simulink model "MPPCMcontrol"  (R2021a)
settings: Solver=FixedStepDiscrete  StartTime=0.0  StopTime=0.0015  FixedStep=2.5e-8  RelTol=1e-3
libraries: modelsimlib x1
settings Model: Creator=xiang  LastModifiedBy=xiang

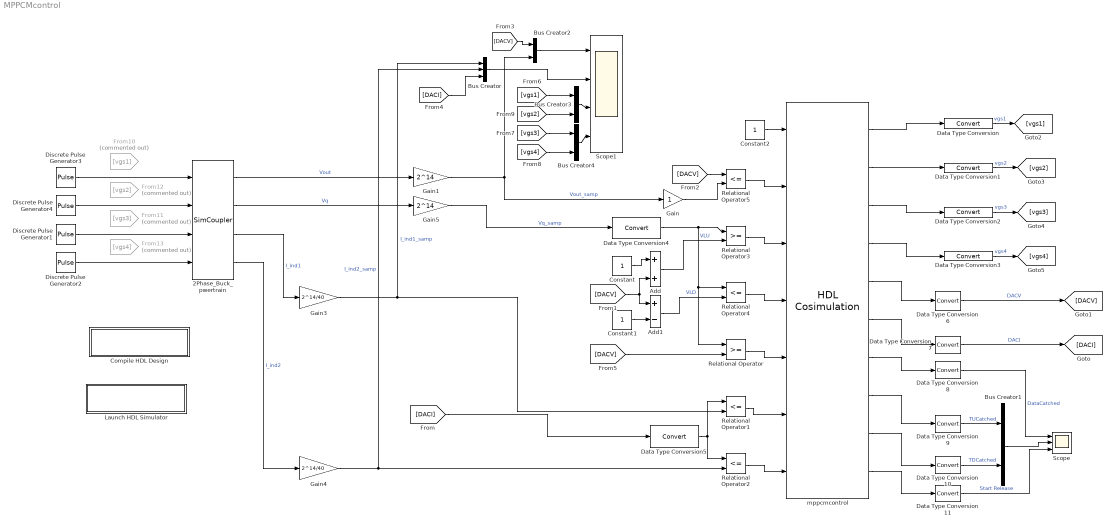
== system MPPCMcontrol ==
  2Phase_Buck_pwertrain : S-Function  FunctionName=SimCoupler  Parameters='C:\Users\xiang\Documents\PSIM\AVP_Simulink_cosim\2Phase_Buck_pwertrain.psimsch;flag_interpolation=0'  SFunctionDeploymentMode=off  EnableBusSupport=off
      mask init:
      | c=[0:10:360]*pi/180;
      | x1=cos(c)*30; y1=sin(c)*30+20;
      | x2=cos(c)*30;y2=sin(c)*30-20;
      settings: OpenFcn=PSimDialog('PSimFileEdt','Value','Parameters');  CloseFcn=close(gcf);
      mask Display: plot(-60,-60,60,60,x1,y1,x2,y2);port_label('input', 1, 'Q11');port_label('input', 2, 'Q12');port_label('input', 3, 'Q13');port_label('input', 4, 'Q14');port_label('output', 1, 'Vout');port_label('output', 2, 'Vq');port_label('output', 3, 'I_ind1');port_label('output', 4, 'I_ind2');
  Add : Sum
  Add1 : Sum  Inputs=+-
  Bus Creator : BusCreator  Inputs=3
  Bus Creator{1..4} (4 alike) : BusCreator  Inputs=2
  Compile HDL Design : Subsystem
      settings: OpenFcn=eval('compile_hdl_design_mppcmcontrol');
      mask Display: disp(['Double-Click to' char(10) 'compile HDL files'])
  Constant : Constant
  Constant1 : Constant
  Constant2 : Constant  OutDataTypeStr=boolean
  Data Type Conversion{,1..11} (12 alike) : DataTypeConversion
  Discrete Pulse Generator1 : DiscretePulseGenerator  Period=200/2.5  PulseWidth=40/2.5  PhaseDelay=100/2.5  SampleTime=2.5e-8
  Discrete Pulse Generator2 : DiscretePulseGenerator  Period=200/2.5  PulseWidth=150/2.5  PhaseDelay=150/2.5  SampleTime=2.5e-8
  Discrete Pulse Generator3 : DiscretePulseGenerator  Period=200/2.5  PulseWidth=40/2.5  SampleTime=2.5e-8
  Discrete Pulse Generator4 : DiscretePulseGenerator  Period=200/2.5  PulseWidth=150/2.5  PhaseDelay=50/2.5  SampleTime=2.5e-8
  From10 : From  Commented=on  GotoTag=vgs1
  From11 : From  Commented=on  GotoTag=vgs3
  From12 : From  Commented=on  GotoTag=vgs2
  From13 : From  Commented=on  GotoTag=vgs4
  Gain : Gain
  Gain1 : Gain  Gain=2^14
  Gain3 : Gain  Gain=2^14/40
  Gain4 : Gain  Gain=2^14/40
  Gain5 : Gain  Gain=2^14
  Launch HDL Simulator : Subsystem
      settings: OpenFcn=eval('launch_hdl_simulator_mppcmcontrol');
      mask Display: disp(['Double-Click to' char(10) 'launch HDL simulator'])
  Relational Operator : RelationalOperator  OutDataTypeStr=boolean  RndMeth=Simplest
  Relational Operator{1..2,4..5} (4 alike) : RelationalOperator  Operator=<=  OutDataTypeStr=boolean  RndMeth=Simplest
  Relational Operator3 : RelationalOperator  OutDataTypeStr=boolean  RndMeth=Simplest
  Scope : Scope  NumInputPorts=3
  Scope1 : Scope  NumInputPorts=4
  mppcmcontrol : modelsimlib/HDL Cosimulation  PortPaths=/mppcmcontrol/resetn;/mppcmcontrol/CompV;/mppcmcontrol/CompVqu;/mppcmcontrol/CompVqd;/mppcmcontrol/CompVq;/mppcmcontrol/CompI3;/mppcmcontrol/CompI4;/mppcmcontrol/PWM1;/mppcmcontrol/PWM2;/mppcmcontrol/PWM3;/mppcmcontrol/PWM4;/mppcmcontrol/DACV;/mppcmcontrol/DACI;/mppcmcontrol/DataCatched;/mppcmcontrol/TUCatched;/mppcmcontrol/TDCatched;/mppcmcontrol/StartReleaseLed  PortModes=[1 1 1 1 1 1 1 2 2 2 2 2 2 2 2 2 2 ]  PortTimes=[-1,-1,-1,-1,-1,-1,-1,2.5e-8,2.5e-8,2.5e-8,2.5e-8,2.5e-8,2.5e-8,2.5e-8,2.5e-8,2.5e-8,2.5e-8]  PortSigns=[-1 -1 -1 -1 -1 -1 -1 -1 -1 -1 -1 -1 -1 -1 -1 -1 -1 ]  PortFracLengths=[0,0,0,0,0,0,0,0,0,0,0,0,0,0,0,0,0]  CommLocal=on  CommSharedMemory=on  CommPortNumber=4449  CommShowInfo=on  ClockModes=[]  ClockTimes=[]  TclPreSimCommand=|  TclPostSimCommand=|  TimingMode=s  TimingScaleFactor=1  idxCellArray={'UNUSED_VAR'}  CosimBypass=Full Simulation  AllowDirectFeedthrough=on  ProductName=EDA Simulator Link MQ  RunAutoTimescale=off  HdlClocks=/mppcmcontrol/CLK 25 ns;  PreRunTime=0  PreRunTimeUnit=ns
      TclPreSimCommand=|
      | force /mppcmcontrol/CLK 0 0 ns, 1 12.5 ns -repeat 25 ns;
      | force /mppcmcontrol/resetn 0 0 ns, 1 5 ns;
      TclPostSimCommand=|
      | noforce /mppcmcontrol/CLK;
      | puts "done";
      settings: SourceProductBaseCode=ES
  wires:
  Add1/1 -> Relational Operator4/2  "VLD"
  mppcmcontrol/6 -> Data Type Conversion7/1
  Relational Operator3/1 -> mppcmcontrol/3
  Relational Operator2/1 -> mppcmcontrol/7
  Data Type Conversion4/1 -> Relational Operator/1, Relational Operator4/1, Relational Operator3/1
  Relational Operator1/1 -> mppcmcontrol/6
  mppcmcontrol/5 -> Data Type Conversion6/1
  mppcmcontrol/2 -> Data Type Conversion1/1
  Relational Operator4/1 -> mppcmcontrol/4
  mppcmcontrol/3 -> Data Type Conversion2/1
  mppcmcontrol/8 -> Data Type Conversion9/1
  Relational Operator/1 -> mppcmcontrol/5
  Relational Operator5/1 -> mppcmcontrol/2
  Gain/1 -> Relational Operator5/2
  Constant1/1 -> Add1/2
  Add/1 -> Relational Operator3/2  "VLU"
  Constant/1 -> Add/1
  mppcmcontrol/4 -> Data Type Conversion3/1
  mppcmcontrol/7 -> Data Type Conversion8/1
  mppcmcontrol/9 -> Data Type Conversion10/1
  Bus Creator1/1 -> Scope/2
  mppcmcontrol/1 -> Data Type Conversion/1
  Data Type Conversion5/1 -> Relational Operator2/1, Relational Operator1/1
  Constant2/1 -> mppcmcontrol/1
  Data Type Conversion7/1 -> [DACI]  "DACI"
  Data Type Conversion6/1 -> [DACV]  "DACV"
  [DACI] -> Data Type Conversion5/1
  [DACV] -> Add/2, Add1/1
  2Phase_Buck_pwertrain/2 -> Gain5/1  "Vq"
  2Phase_Buck_pwertrain/1 -> Gain1/1  "Vout"
  [DACV] -> Relational Operator5/1
  2Phase_Buck_pwertrain/3 -> Gain3/1  "I_ind1"
  2Phase_Buck_pwertrain/4 -> Gain4/1  "I_ind2"
  Bus Creator/1 -> Scope1/2
  [DACI] -> Bus Creator/3
  [DACV] -> Relational Operator/2
  [DACV] -> Bus Creator2/1
  Bus Creator2/1 -> Scope1/1
  Gain3/1 -> Bus Creator/1, Relational Operator1/2  "I_ind1_samp"
  Gain4/1 -> Bus Creator/2, Relational Operator2/2  "I_ind2_samp"
  Data Type Conversion/1 -> [vgs1]  "vgs1"
  Data Type Conversion1/1 -> [vgs2]  "vgs2"
  Data Type Conversion2/1 -> [vgs3]  "vgs3"
  Data Type Conversion3/1 -> [vgs4]  "vgs4"
  [vgs1] -> Bus Creator3/1
  [vgs3] -> Bus Creator4/1
  [vgs4] -> Bus Creator4/2
  [vgs2] -> Bus Creator3/2
  Bus Creator3/1 -> Scope1/3
  Bus Creator4/1 -> Scope1/4
  Gain1/1 -> Gain/1, Bus Creator2/2  "Vout_samp"
  Gain5/1 -> Data Type Conversion4/1  "Vq_samp"
  Data Type Conversion8/1 -> Scope/1  "DataCatched"
  Data Type Conversion9/1 -> Bus Creator1/1  "TUCatched"
  Data Type Conversion10/1 -> Bus Creator1/2  "TDCatched"
  mppcmcontrol/10 -> Data Type Conversion11/1
  Discrete Pulse Generator3/1 -> 2Phase_Buck_pwertrain/1
  Discrete Pulse Generator4/1 -> 2Phase_Buck_pwertrain/2
  Discrete Pulse Generator1/1 -> 2Phase_Buck_pwertrain/3
  Discrete Pulse Generator2/1 -> 2Phase_Buck_pwertrain/4
  Data Type Conversion11/1 -> Scope/3  "Start Release"

== system MPPCMcontrol/Compile HDL Design ==

== system MPPCMcontrol/Launch HDL Simulator ==
